simulink library "bluetooth_lib"  (Simulink 6.0)
settings: Solver=ode45  SolverMode=SingleTasking  StartTime=0.0  StopTime=10.0  RelTol=1e-3
undefined symbols (not defined in the file or in its folder): awgn_802_seed, fixed_hop_freq, hop_seed, rate_802_seed
libraries: dspindex x12, commutil2 x12, dspsrcs4 x9, bluetooth_lib x7, dspsigattribs x3, dsparch4 x2, dspsigops x2, commdigbbndfm2 x1, dspstat3 x1, dspbuff3 x1, simulink3 x1
settings Model: Creator=stuartm  LastModifiedBy=mmclerno  ProdHWDeviceType=Specified
settings DataIOCC: SignalLoggingName=logsOut
settings OptimizationCC: BooleanDataType=off
settings DebuggingCC: CheckExecutionContextPreStartOutputMsg=on  CheckExecutionContextRuntimeOutputMsg=on  SolverPrmCheckMsg=none
settings HardwareCC: ProdHWDeviceType=Specified

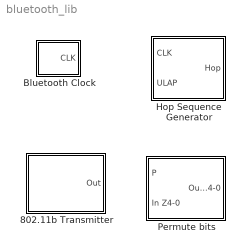
== system bluetooth_lib ==
  802.11b Transmitter : Subsystem  PropExecContextAcrossSSBoundary=on  mask{On=on, rate=200, m=1e-3, v=0, power=0.1, Freq_Number=39, rate_seed=rate_802_seed, awgn_seed=awgn_802_seed}
      mask prompts: On "Turn On 802.11"; rate "Average Rate (1/sec) (999 for constant)"; m "Mean Length (secs)"; v "Length Variance (sec^2)"; Freq_Number "Frequency Number (0-78)"; rate_seed "Rate Seed"; awgn_seed "Noise seed"
      mask init:
      | if On==1
      |    str='On';
      | else
      |   str='Off';
      | end;
      | 
      | adjusted_rate=rate/(1-rate*m); % account for finite packet length reducing rate
      mask Display: disp(['802.11b\nInterferer\n' str])
  Bluetooth Clock : Subsystem  PropExecContextAcrossSSBoundary=on  mask(Bluetooth Clock){Ts=(1/1600)/2}
      mask prompts: Ts "Sample Time"
  Hop Sequence Generator : Subsystem  PropExecContextAcrossSSBoundary=on  mask(Hop Sequence Generator){Hop_Mode=Connection State Hop Sequence, hop_seed=hop_seed, fixed_hop_freq=fixed_hop_freq}
      mask prompts: Hop_Mode "Hop mode"; hop_seed "Hop seed (for white random sequence option)"; fixed_hop_freq "Fixed hop frequency (for fixed option)"
      mask help: Generate a sequence of hop frequencies in the range 0 to 78. Can generate either the connection state hop sequence, a random white sequence, or be fixed.
      mask StyleString: popup(Connection State Hop Sequence|Random White Hop Sequence|Fixed Frequency),edit,edit
  Permute bits : Subsystem  PropExecContextAcrossSSBoundary=on  mask{P=[13 12], First=[1 2], Second=[0 3]}
      mask prompts: P "P bit pair"; First "Pair of bits that first P bit switches"; Second "Pair of bits that second P bit switches"
      mask Display: disp(['P' num2str(P(1)) ': {Z' num2str(First(1)) ',Z' num2str(First(2)) '}\n'  'P' num2str(P(2)) ': {Z' num2str(Second(1)) ',Z' num2str(Second(2)) '}'])

== system bluetooth_lib/802.11b Transmitter ==
  1/100packet resolution : ZeroOrderHold  SampleTime=(1/1600)/100
  22MHz noise in 100MHz signal : Subsystem  TreatAsAtomicUnit=on  PropExecContextAcrossSSBoundary=on
  Buffer to same frame-size as channel : dspbuff3/Buffer  N=62500  V=0  ic=0
  Enable control : Subsystem  PropExecContextAcrossSSBoundary=on
      mask Display:
      | disp('Enable\n
      | Logic')
  Square pulse with Poisson process : Subsystem  PropExecContextAcrossSSBoundary=on  mask(Poisson process){rate=adjusted_rate, m=m, v=v, seed=rate_seed}
      mask prompts: rate "Average Rate (1/sec)"; m "Mean Length"; v "Length Variance"
      mask Display: plot(exp(-(0:.4:3)))
  Out : Outport
  tag scope: Packet_Envelope_802=global
  wires:
  Enable control/1(Out) -> 22MHz noise in 100MHz signal/Enable
  Square pulse with Poisson process/1(hit) -> [Packet_Envelope_802], 1/100packet resolution/1
  1/100packet resolution/1 -> Enable control/1(In)
  Buffer to same frame-size as channel/1 -> Out/1
  22MHz noise in 100MHz signal/1(Out) -> Buffer to same frame-size as channel/1

== system bluetooth_lib/Bluetooth Clock ==
  DSP Constant : dspsrcs4/DSP Constant  Value=1  SampleMode=Discrete  discreteOutput=Sample-based  continuousOutput=Sample-based  sampTime=Ts  framePeriod=Ts  dataType=Inherit from 'Constant value'  wordLen=16  udDataType=sfix(16)  fracBitsMode=Best precision  numFracBits=15  InterpretAs1D=off  Ts=Ts  FramebasedOutput=off
  Delay : dspsigops/Delay  dly_unit=Samples  delay=1  ic_detail=off  dif_ic_for_ch=off  dif_ic_for_dly=off  ic=0  reset_popup=None
  Sum : Sum  Inputs=|++  SaturateOnIntegerOverflow=on  InputSameDT=on
  CLK : Outport
  wires:
  Sum/1 -> Delay/1
  DSP Constant/1 -> Sum/1
  Delay/1 -> Sum/2, CLK/1

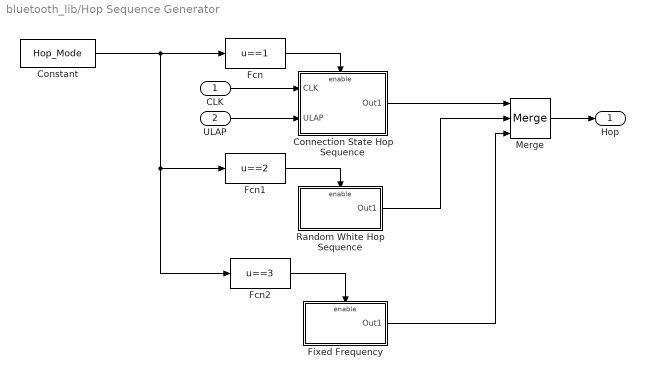
== system bluetooth_lib/Hop Sequence Generator ==
  CLK : Inport  LatchInput=off
  ULAP : Inport  Port=2  LatchInput=off
  Connection State Hop Sequence : Subsystem  TreatAsAtomicUnit=on  PropExecContextAcrossSSBoundary=on
  Constant : Constant  Value=Hop_Mode
  Fcn : Fcn  Expr=u==1
  Fcn1 : Fcn  Expr=u==2
  Fcn2 : Fcn  Expr=u==3
  Fixed Frequency : Subsystem  TreatAsAtomicUnit=on  PropExecContextAcrossSSBoundary=on
  Merge : Merge  Inputs=3
  Random White Hop Sequence : Subsystem  TreatAsAtomicUnit=on  PropExecContextAcrossSSBoundary=on
  Hop : Outport
  wires:
  ULAP/1 -> Connection State Hop Sequence/2(ULAP)
  CLK/1 -> Connection State Hop Sequence/1(CLK)
  Constant/1 -> Fcn/1, Fcn1/1, Fcn2/1
  Merge/1 -> Hop/1
  Connection State Hop Sequence/1(Out1) -> Merge/1
  Random White Hop Sequence/1(Out1) -> Merge/2
  Fixed Frequency/1(Out1) -> Merge/3
  Fcn/1 -> Connection State Hop Sequence/Enable
  Fcn1/1 -> Random White Hop Sequence/Enable
  Fcn2/1 -> Fixed Frequency/Enable

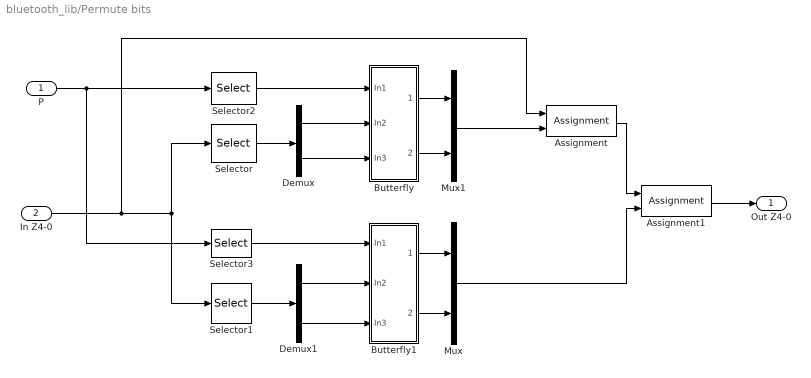
== system bluetooth_lib/Permute bits ==
  P : Inport  LatchInput=off
  In Z4-0 : Inport  Port=2  LatchInput=off
  Assignment : Assignment  Elements=[First(1) First(2)] +1
  Assignment1 : Assignment  Elements=[Second(1) Second(2)] +1
  Butterfly : Subsystem  PropExecContextAcrossSSBoundary=on
  Butterfly1 : Subsystem  PropExecContextAcrossSSBoundary=on
  Demux : Demux  Outputs=2
  Demux1 : Demux  Outputs=2
  Mux : Mux  Inputs=2
  Mux1 : Mux  Inputs=2
  Selector : Selector  Elements=[First(1) First(2)] +1  InputPortWidth=5
  Selector1 : Selector  Elements=[Second(1) Second(2)] +1  InputPortWidth=5
  Selector2 : Selector  Elements=[P(1)] +1  InputPortWidth=14
  Selector3 : Selector  Elements=[P(2)] +1  InputPortWidth=14
  Out Z4-0 : Outport
  wires:
  Demux1/2 -> Butterfly1/3(In3)
  Selector3/1 -> Butterfly1/1(In1)
  Demux/1 -> Butterfly/2(In2)
  Butterfly/1(Out1) -> Mux1/1
  Butterfly1/1(Out1) -> Mux/1
  Butterfly1/2(Out2) -> Mux/2
  Mux/1 -> Assignment1/2
  In Z4-0/1 -> Selector/1, Selector1/1, Assignment/1
  Selector/1 -> Demux/1
  Selector1/1 -> Demux1/1
  Butterfly/2(Out2) -> Mux1/2
  Mux1/1 -> Assignment/2
  Assignment/1 -> Assignment1/1
  Assignment1/1 -> Out Z4-0/1
  Demux/2 -> Butterfly/3(In3)
  Demux1/1 -> Butterfly1/2(In2)
  P/1 -> Selector2/1, Selector3/1
  Selector2/1 -> Butterfly/1(In1)

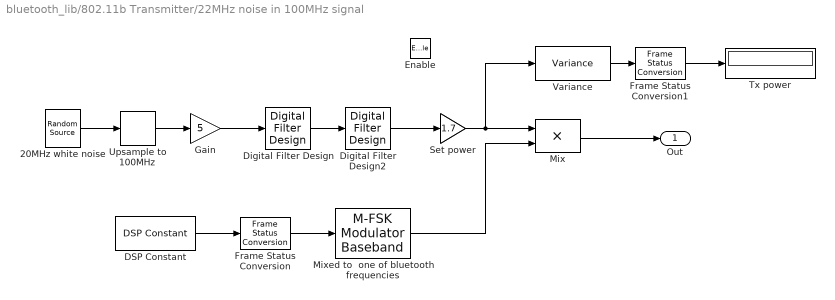
== system bluetooth_lib/802.11b Transmitter/22MHz noise in 100MHz signal ==
  Enable : EnablePort
  20MHz white noise : dspsrcs4/Random Source  SrcType=Gaussian  NormMethod=Ziggurat  CltLength=12  Min=0  Max=1  Mean=0  Var=power  RepMode=Specify seed  rawSeed=awgn_seed  Inherit=off  SampMode=Discrete  SampTime=1/20e6  SampFrame=62500/500  DataType=Double  OutComplex=Complex
  DSP Constant : dspsrcs4/DSP Constant  Value=Freq_Number  SampleMode=Discrete  discreteOutput=Sample-based  continuousOutput=Sample-based  sampTime=.01/1600  framePeriod=.01/1600  dataType=Inherit from 'Constant value'  isSigned=on  wordLen=16  udDataType=sfix(16)  fracBitsMode=Best precision  numFracBits=15  InterpretAs1D=off  Ts=.01/1600  FramebasedOutput=off
  Digital Filter Design : dsparch4/Digital Filter Design
  Digital Filter Design2 : dsparch4/Digital Filter Design
  Frame Status Conversion : dspsigattribs/Frame Status Conversion  growRefPort=off  outframe=Frame-based
  Frame Status Conversion1 : dspsigattribs/Frame Status Conversion  growRefPort=off  outframe=Sample-based
  Gain : Gain  Gain=5  SaturateOnIntegerOverflow=on
  Mix : Product  SaturateOnIntegerOverflow=on  InputSameDT=on
  "Mixed to  one of bluetooth frequencies " : commdigbbndfm2/M-FSK Modulator Baseband  M=79  InType=Integer  Enc=Binary  freqSep=1e6  phaseType=Continuous  numSamp=6.25e4/100
  Set power : Gain  Gain=1.7  SaturateOnIntegerOverflow=on
  Tx power : Display
  Upsample to 100MHz : dspsigops/Upsample  N=5  phase=0  ic=0  mode=Maintain input frame rate
  Variance : dspstat3/Variance  DialogController=dspDDGCreate  DialogControllerArgs=DataTag3  run=off  reset_popup=None  roundingMode=Floor  overflowMode=off
  Out : Outport  OutputWhenDisabled=reset  InitialOutput=0
  wires:
  Digital Filter Design/1 -> Digital Filter Design2/1
  Digital Filter Design2/1 -> Set power/1
  Set power/1 -> Variance/1, Mix/1
  Frame Status Conversion1/1 -> Tx power/1
  Variance/1 -> Frame Status Conversion1/1
  Gain/1 -> Digital Filter Design/1
  DSP Constant/1 -> Frame Status Conversion/1
  "Mixed to  one of bluetooth frequencies "/1 -> Mix/2
  Frame Status Conversion/1 -> "Mixed to  one of bluetooth frequencies "/1
  20MHz white noise/1 -> Upsample to 100MHz/1
  Mix/1 -> Out/1
  Upsample to 100MHz/1 -> Gain/1

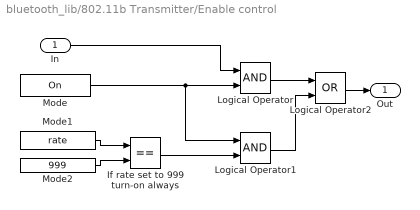
== system bluetooth_lib/802.11b Transmitter/Enable control ==
  In : Inport  LatchInput=off
  If rate set to 999 turn-on always : RelationalOperator  Operator===  InputSameDT=on
  Logical Operator : Logic
  Logical Operator1 : Logic
  Logical Operator2 : Logic  Operator=OR
  Mode : Constant  Value=On
  Mode1 : Constant  Value=rate
  Mode2 : Constant  Value=999
  Out : Outport
  wires:
  Logical Operator2/1 -> Out/1
  In/1 -> Logical Operator/1
  Logical Operator1/1 -> Logical Operator2/2
  Mode/1 -> Logical Operator1/1, Logical Operator/2
  Logical Operator/1 -> Logical Operator2/1
  If rate set to 999 turn-on always/1 -> Logical Operator1/2
  Mode1/1 -> If rate set to 999 turn-on always/1
  Mode2/1 -> If rate set to 999 turn-on always/2

== system bluetooth_lib/802.11b Transmitter/Square pulse with Poisson process ==
  S-Function1 : S-Function  FunctionName=bluetooth_poissonevent  Parameters=adjusted_rate,m,v,seed
  hit : Outport  InitialOutput=0
  wires:
  S-Function1/1 -> hit/1

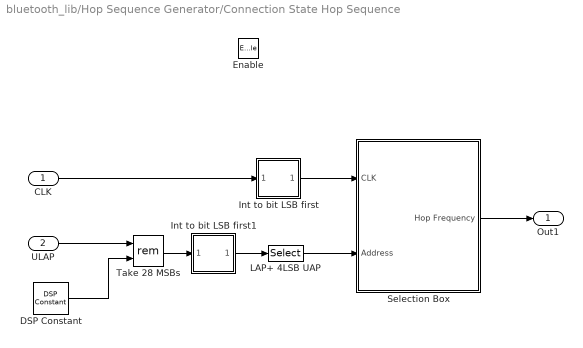
== system bluetooth_lib/Hop Sequence Generator/Connection State Hop Sequence ==
  CLK : Inport  LatchInput=off
  ULAP : Inport  Port=2  LatchInput=off
  Enable : EnablePort
  DSP Constant : dspsrcs4/DSP Constant  Value=2^28  InterpretAs1D=off  SampleMode=Discrete  Ts=(1/1600)/2  FramebasedOutput=off
  Int to bit LSB first : Subsystem  PropExecContextAcrossSSBoundary=on  mask{Numbits=28}
      mask prompts: Numbits "Number of bits"
      mask Display:
      | disp('Int to bit\n
      | LSB first');
  Int to bit LSB first1 : Subsystem  PropExecContextAcrossSSBoundary=on  mask{Numbits=28}
      mask prompts: Numbits "Number of bits"
      mask Display:
      | disp('Int to bit\n
      | LSB first');
  LAP+ 4LSB UAP : Selector  Elements=[0:27] +1  InputPortWidth=28
  Selection Box : Subsystem  PropExecContextAcrossSSBoundary=on
  Take 28 MSBs : Math  Operator=rem  SaturateOnIntegerOverflow=on
  Out1 : Outport
  wires:
  ULAP/1 -> Take 28 MSBs/1
  Take 28 MSBs/1 -> Int to bit LSB first1/1(In1)
  DSP Constant/1 -> Take 28 MSBs/2
  CLK/1 -> Int to bit LSB first/1(In1)
  Int to bit LSB first/1(Out1) -> Selection Box/1(CLK)
  Int to bit LSB first1/1(Out1) -> LAP+ 4LSB UAP/1
  LAP+ 4LSB UAP/1 -> Selection Box/2(Address)
  Selection Box/1(Hop Frequency) -> Out1/1

== system bluetooth_lib/Hop Sequence Generator/Fixed Frequency ==
  Enable : EnablePort
  A fixed hop frequency : dspsrcs4/DSP Constant  Value=fixed_hop_freq  SampleMode=Discrete  discreteOutput=Sample-based (interpret vectors as 1-D)  continuousOutput=Sample-based  sampTime=(1/1600)/2  framePeriod=(1/1600)/2  dataType=Inherit from 'Constant value'  isSigned=on  wordLen=16  udDataType=sfix(16)  fracBitsMode=Best precision  numFracBits=15  InterpretAs1D=on  Ts=(1/1600)/2  FramebasedOutput=off
  Out1 : Outport  InitialOutput=fixed_hop_freq
  wires:
  A fixed hop frequency/1 -> Out1/1

== system bluetooth_lib/Hop Sequence Generator/Random White Hop Sequence ==
  Enable : EnablePort
  Frequency hopping code 1/1600 sec (page 127) : Subsystem  PropExecContextAcrossSSBoundary=on  mask(Random-Integer Generator){mul=79, seed=hop_seed, Ts=(1/1600)/2, frameBased=off, sampPerFrame=1, orient=off}
      mask prompts: mul "M-ary number:"; seed "Initial seed:"; Ts "Sample time:"; frameBased "Frame-based outputs"; sampPerFrame "Samples per frame:"; orient "Interpret vector parameters as 1-D"
      mask help: Generate integers randomly distributed in range [0, M-1], where M is the M-ary number.
      mask init:
      | if (frameBased & sampPerFrame > 1), dsp_sampFrame = sampPerFrame;
      | else dsp_sampFrame = 1; end
      | eStr=commblkrandintsrc2(gcb,'init');
      | if(eStr.ecode==1)
      |     error(eStr.emsg);
      | end
      mask Help: helpview(commbhelp)
      mask CallbackString: |||commblkrandintsrc2(gcb,'cbFrameBased');||commblkrandintsrc2(gcb,'cbOrient');
      mask Display: disp('Random int')
  Out1 : Outport
  wires:
  Frequency hopping code 1/1600 sec (page 127)/1(out_1) -> Out1/1

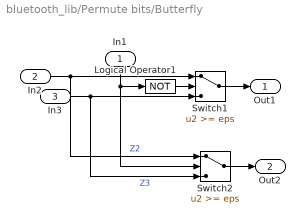
== system bluetooth_lib/Permute bits/Butterfly ==
  In1 : Inport  Orientation=down  LatchInput=off
  In2 : Inport  Port=2  LatchInput=off
  In3 : Inport  Port=3  LatchInput=off
  Logical Operator1 : Logic  Operator=NOT
  Switch1 : Switch  Threshold=eps  SaturateOnIntegerOverflow=on  InputSameDT=on
  Switch2 : Switch  Threshold=eps  SaturateOnIntegerOverflow=on  InputSameDT=on
  Out1 : Outport
  Out2 : Outport  Port=2
  wires:
  Switch2/1 -> Out2/1
  Switch1/1 -> Out1/1
  Logical Operator1/1 -> Switch1/2
  In1/1 -> Switch2/2, Logical Operator1/1
  In3/1 -> Switch1/3, Switch2/3  "Z3"
  In2/1 -> Switch1/1, Switch2/1  "Z2"

== system bluetooth_lib/Permute bits/Butterfly1 ==
  In1 : Inport  Orientation=down  LatchInput=off
  In2 : Inport  Port=2  LatchInput=off
  In3 : Inport  Port=3  LatchInput=off
  Logical Operator1 : Logic  Operator=NOT
  Switch1 : Switch  Threshold=eps  SaturateOnIntegerOverflow=on  InputSameDT=on
  Switch2 : Switch  Threshold=eps  SaturateOnIntegerOverflow=on  InputSameDT=on
  Out1 : Outport
  Out2 : Outport  Port=2
  wires:
  In2/1 -> Switch2/1, Switch1/1  "Z2"
  In3/1 -> Switch2/3, Switch1/3  "Z3"
  In1/1 -> Logical Operator1/1, Switch2/2
  Logical Operator1/1 -> Switch1/2
  Switch1/1 -> Out1/1
  Switch2/1 -> Out2/1

== system bluetooth_lib/Hop Sequence Generator/Connection State Hop Sequence/Int to bit LSB first ==
  In1 : Inport  LatchInput=off
  Flip : dspindex/Flip  dim=Columns
  Integer to Bit Converter3 : commutil2/Integer to Bit Converter  nbits=Numbits
  Out1 : Outport
  wires:
  Integer to Bit Converter3/1 -> Flip/1
  Flip/1 -> Out1/1
  In1/1 -> Integer to Bit Converter3/1

== system bluetooth_lib/Hop Sequence Generator/Connection State Hop Sequence/Int to bit LSB first1 ==
  In1 : Inport  LatchInput=off
  Flip : dspindex/Flip  dim=Columns
  Integer to Bit Converter3 : commutil2/Integer to Bit Converter  nbits=Numbits
  Out1 : Outport
  wires:
  In1/1 -> Integer to Bit Converter3/1
  Flip/1 -> Out1/1
  Integer to Bit Converter3/1 -> Flip/1

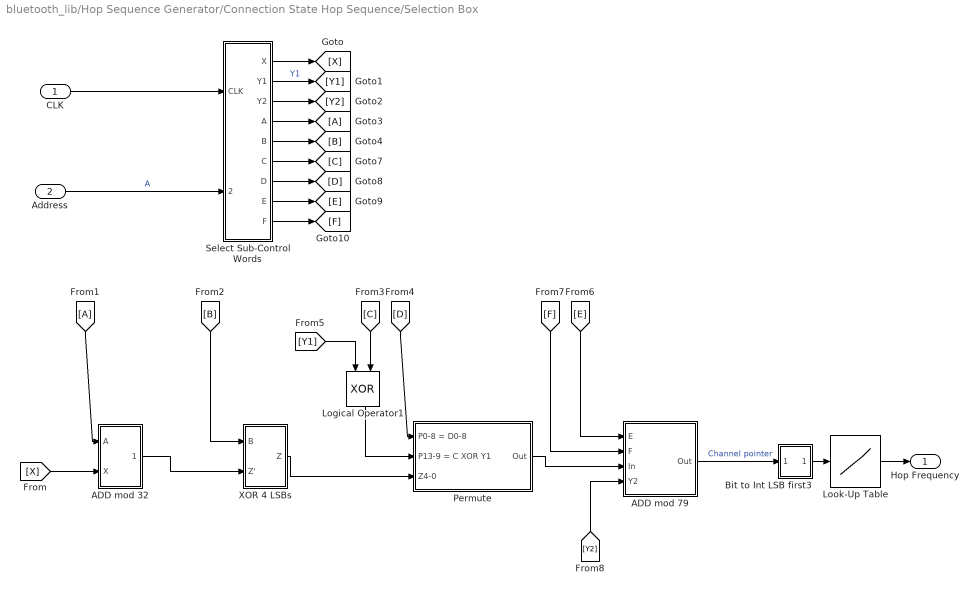
== system bluetooth_lib/Hop Sequence Generator/Connection State Hop Sequence/Selection Box ==
  CLK : Inport  LatchInput=off
  Address : Inport  Port=2  LatchInput=off
  ADD mod 32 : Subsystem  PropExecContextAcrossSSBoundary=on
  ADD mod 79 : Subsystem  PropExecContextAcrossSSBoundary=on
  Bit to Int LSB first3 : Subsystem  PropExecContextAcrossSSBoundary=on  mask{Numbits=7}
      mask prompts: Numbits "Number of bits"
      mask Display:
      | disp('Bit to Int\n
      | LSB first');
  Logical Operator1 : Logic  Orientation=down  Operator=XOR
  Look-Up Table : Lookup  DialogController=Simulink.DDGSource  InputValues=0:78  OutputValues=[0:2:78 1:2:77]  SaturateOnIntegerOverflow=on
  Permute : Subsystem  PropExecContextAcrossSSBoundary=on
  Select Sub-Control Words : Subsystem  PropExecContextAcrossSSBoundary=on
  XOR 4 LSBs : Subsystem  PropExecContextAcrossSSBoundary=on
  Hop Frequency : Outport
  wires:
  [A] -> ADD mod 32/1(A)
  [B] -> XOR 4 LSBs/1(B)
  Logical Operator1/1 -> Permute/2(P13-9 = C XOR Y1)
  [D] -> Permute/1(P0-8 = D0-8)
  Permute/1(Out) -> ADD mod 79/3(In)
  [C] -> Logical Operator1/2
  [Y1] -> Logical Operator1/1
  [E] -> ADD mod 79/1(E)
  [F] -> ADD mod 79/2(F)
  [Y2] -> ADD mod 79/4(Y2)
  ADD mod 79/1(Out) -> Bit to Int LSB first3/1(In1)  "Channel pointer"
  XOR 4 LSBs/1(Z) -> Permute/3(Z4-0)
  Look-Up Table/1 -> Hop Frequency/1
  CLK/1 -> Select Sub-Control Words/1(CLK)
  Select Sub-Control Words/1(X) -> [X]
  Select Sub-Control Words/3(Y2) -> [Y2]
  Address/1 -> Select Sub-Control Words/2(Address)  "A"
  Select Sub-Control Words/4(A) -> [A]
  Select Sub-Control Words/5(B) -> [B]
  Select Sub-Control Words/6(C) -> [C]
  Select Sub-Control Words/7(D) -> [D]
  Select Sub-Control Words/8(E) -> [E]
  Select Sub-Control Words/9(F) -> [F]
  Select Sub-Control Words/2(Y1) -> [Y1]  "Y1"
  [X] -> ADD mod 32/2(X)
  ADD mod 32/1(Out1) -> XOR 4 LSBs/2(Z')
  Bit to Int LSB first3/1(Out1) -> Look-Up Table/1

== system bluetooth_lib/Hop Sequence Generator/Random White Hop Sequence/Frequency hopping code 1/1600 sec (page 127) ==
  Frame Status Conversion : dspsigattribs/Frame Status Conversion  growRefPort=off  outframe=Sample-based
  Random Source : dspsrcs4/Random Source  SrcType=Uniform  Min=-1+eps  Max=mul-1  Mean=0  Var=1  RepMode=Specify seed  Seed=seed  Inherit=off  SampMode=Discrete  SampTime=Ts  SampFrame=dsp_sampFrame  OutComplex=Real
  Reshape : simulink3/Signals & Systems/Reshape  OutputDimensionality=1-D array  OutputDimensions=[sampPerFrame,max([length(mul), length(seed)])]
  Rounding Function : Rounding  Operator=ceil
  out_1 : Outport  InitialOutput=0
  wires:
  Frame Status Conversion/1 -> Reshape/1
  Random Source/1 -> Rounding Function/1
  Reshape/1 -> out_1/1
  Rounding Function/1 -> Frame Status Conversion/1

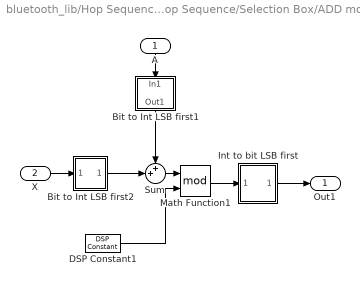
== system bluetooth_lib/Hop Sequence Generator/Connection State Hop Sequence/Selection Box/ADD mod 32 ==
  A : Inport  Orientation=down  LatchInput=off
  X : Inport  Port=2  LatchInput=off
  Bit to Int LSB first1 : Subsystem  Orientation=down  PropExecContextAcrossSSBoundary=on  mask{Numbits=5}
      mask prompts: Numbits "Number of bits"
      mask Display:
      | disp('Bit to Int\n
      | LSB first');
  Bit to Int LSB first2 : Subsystem  PropExecContextAcrossSSBoundary=on  mask{Numbits=5}
      mask prompts: Numbits "Number of bits"
      mask Display:
      | disp('Bit to Int\n
      | LSB first');
  DSP Constant1 : dspsrcs4/DSP Constant  Value=32  InterpretAs1D=off  SampleMode=Discrete  Ts=(1/1600)/2  FramebasedOutput=off
  Int to bit LSB first : Subsystem  PropExecContextAcrossSSBoundary=on  mask{Numbits=5}
      mask prompts: Numbits "Number of bits"
      mask Display:
      | disp('Int to bit\n
      | LSB first');
  Math Function1 : Math  Operator=mod  SaturateOnIntegerOverflow=on
  Sum : Sum  Inputs=++|  SaturateOnIntegerOverflow=on  InputSameDT=on
  Out1 : Outport
  wires:
  Bit to Int LSB first2/1(Out1) -> Sum/2
  Bit to Int LSB first1/1(Out1) -> Sum/1
  Math Function1/1 -> Int to bit LSB first/1(In1)
  Sum/1 -> Math Function1/1
  DSP Constant1/1 -> Math Function1/2
  A/1 -> Bit to Int LSB first1/1(In1)
  X/1 -> Bit to Int LSB first2/1(In1)
  Int to bit LSB first/1(Out1) -> Out1/1

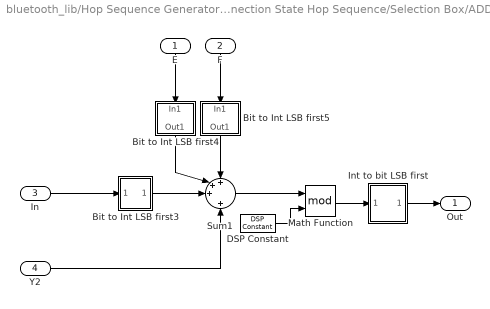
== system bluetooth_lib/Hop Sequence Generator/Connection State Hop Sequence/Selection Box/ADD mod 79 ==
  E : Inport  Orientation=down  LatchInput=off
  F : Inport  Orientation=down  Port=2  LatchInput=off
  In : Inport  Port=3  LatchInput=off
  Y2 : Inport  Port=4  LatchInput=off
  Bit to Int LSB first3 : Subsystem  PropExecContextAcrossSSBoundary=on  mask{Numbits=5}
      mask prompts: Numbits "Number of bits"
      mask Display:
      | disp('Bit to Int\n
      | LSB first');
  Bit to Int LSB first4 : Subsystem  Orientation=down  PropExecContextAcrossSSBoundary=on  mask{Numbits=7}
      mask prompts: Numbits "Number of bits"
      mask Display:
      | disp('Bit to Int\n
      | LSB first');
  Bit to Int LSB first5 : Subsystem  Orientation=down  PropExecContextAcrossSSBoundary=on  mask{Numbits=7}
      mask prompts: Numbits "Number of bits"
      mask Display:
      | disp('Bit to Int\n
      | LSB first');
  DSP Constant : dspsrcs4/DSP Constant  Value=79  InterpretAs1D=off  SampleMode=Discrete  Ts=(1/1600)/2  FramebasedOutput=off
  Int to bit LSB first : Subsystem  PropExecContextAcrossSSBoundary=on  mask{Numbits=7}
      mask prompts: Numbits "Number of bits"
      mask Display:
      | disp('Int to bit\n
      | LSB first');
  Math Function : Math  Operator=mod  SaturateOnIntegerOverflow=on
  Sum1 : Sum  Inputs=+++|+  SaturateOnIntegerOverflow=on  InputSameDT=on
  Out : Outport
  wires:
  Bit to Int LSB first5/1(Out1) -> Sum1/1
  Bit to Int LSB first4/1(Out1) -> Sum1/2
  Sum1/1 -> Math Function/1
  DSP Constant/1 -> Math Function/2
  Bit to Int LSB first3/1(Out1) -> Sum1/3
  E/1 -> Bit to Int LSB first4/1(In1)
  F/1 -> Bit to Int LSB first5/1(In1)
  In/1 -> Bit to Int LSB first3/1(In1)
  Math Function/1 -> Int to bit LSB first/1(In1)
  Y2/1 -> Sum1/4
  Int to bit LSB first/1(Out1) -> Out/1

== system bluetooth_lib/Hop Sequence Generator/Connection State Hop Sequence/Selection Box/Bit to Int LSB first3 ==
  In1 : Inport  LatchInput=off
  Bit to Integer Converter5 : commutil2/Bit to Integer Converter  nbits=Numbits
  Flip1 : dspindex/Flip  dim=Columns
  Out1 : Outport
  wires:
  Flip1/1 -> Bit to Integer Converter5/1
  Bit to Integer Converter5/1 -> Out1/1
  In1/1 -> Flip1/1

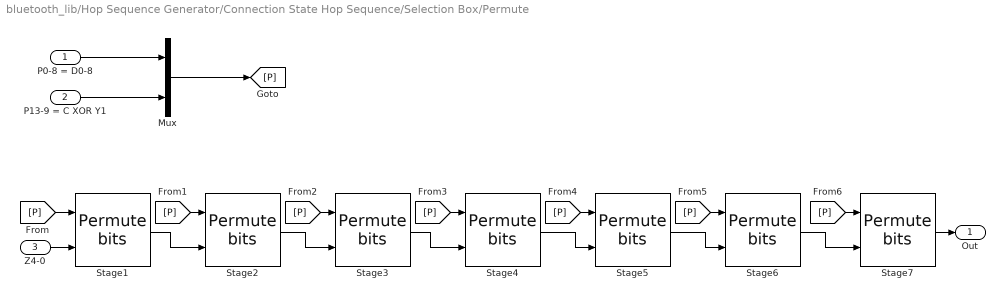
== system bluetooth_lib/Hop Sequence Generator/Connection State Hop Sequence/Selection Box/Permute ==
  P0-8 = D0-8 : Inport  LatchInput=off
  P13-9 = C XOR Y1 : Inport  Port=2  LatchInput=off
  Z4-0 : Inport  Port=3  LatchInput=off
  Mux : Mux  Inputs=2
  Stage1 : bluetooth_lib/Permute bits  P=[13 12]  First=[1 2]  Second=[0 3]
  Stage2 : bluetooth_lib/Permute bits  P=[11 10]  First=[1 3]  Second=[2 4]
  Stage3 : bluetooth_lib/Permute bits  P=[9 8]  First=[0 3]  Second=[1 4]
  Stage4 : bluetooth_lib/Permute bits  P=[7 6]  First=[3 4]  Second=[0 2]
  Stage5 : bluetooth_lib/Permute bits  P=[5 4]  First=[1 3]  Second=[0 4]
  Stage6 : bluetooth_lib/Permute bits  P=[3 2]  First=[3 4]  Second=[1 2]
  Stage7 : bluetooth_lib/Permute bits  P=[1 0]  First=[2 3]  Second=[0 1]
  Out : Outport
  wires:
  Z4-0/1 -> Stage1/2
  Stage1/1 -> Stage2/2
  Mux/1 -> [P]
  [P] -> Stage1/1
  Stage2/1 -> Stage3/2
  [P] -> Stage3/1
  Stage3/1 -> Stage4/2
  [P] -> Stage4/1
  [P] -> Stage5/1
  Stage4/1 -> Stage5/2
  [P] -> Stage6/1
  Stage5/1 -> Stage6/2
  [P] -> Stage7/1
  Stage6/1 -> Stage7/2
  Stage7/1 -> Out/1
  P13-9 = C XOR Y1/1 -> Mux/2
  P0-8 = D0-8/1 -> Mux/1
  [P] -> Stage2/1

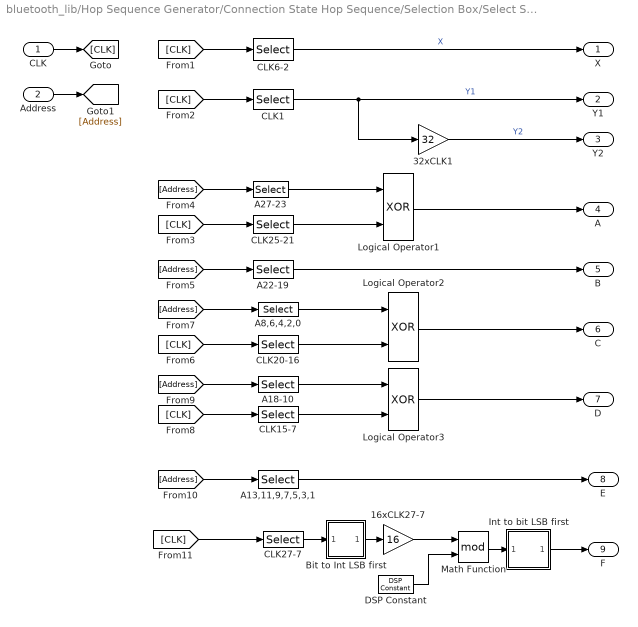
== system bluetooth_lib/Hop Sequence Generator/Connection State Hop Sequence/Selection Box/Select Sub-Control Words ==
  CLK : Inport  LatchInput=off
  Address : Inport  Port=2  LatchInput=off
  16xCLK27-7 : Gain  Gain=16  SaturateOnIntegerOverflow=on
  32xCLK1 : Gain  Gain=32  SaturateOnIntegerOverflow=on
  A13,11,9,7,5,3,1 : Selector  Elements=[1 3 5 7 9 11 13] +1  InputPortWidth=28
  A18-10 : Selector  Elements=[10:18] +1  InputPortWidth=28
  A22-19 : Selector  Elements=[19:22] +1  InputPortWidth=28
  A27-23 : Selector  Elements=[23:27] +1  InputPortWidth=28
  A8,6,4,2,0 : Selector  Elements=[0 2 4 6 8] +1  InputPortWidth=28
  Bit to Int LSB first : Subsystem  PropExecContextAcrossSSBoundary=on  mask{Numbits=21}
      mask prompts: Numbits "Number of bits"
      mask Display:
      | disp('Bit to Int\n
      | LSB first');
  CLK1 : Selector  Elements=[1] +1  InputPortWidth=28
  CLK15-7 : Selector  Elements=[7:15] +1  InputPortWidth=28
  CLK20-16 : Selector  Elements=[16:20] +1  InputPortWidth=28
  CLK25-21 : Selector  Elements=[21:25] +1  InputPortWidth=28
  CLK27-7 : Selector  Elements=[7:27] +1  InputPortWidth=28
  CLK6-2 : Selector  Elements=[2:6] +1  InputPortWidth=28
  DSP Constant : dspsrcs4/DSP Constant  Value=79  InterpretAs1D=off  SampleMode=Discrete  Ts=(1/1600)/2  FramebasedOutput=off
  Int to bit LSB first : Subsystem  PropExecContextAcrossSSBoundary=on  mask{Numbits=7}
      mask prompts: Numbits "Number of bits"
      mask Display:
      | disp('Int to bit\n
      | LSB first');
  Logical Operator1 : Logic  Operator=XOR
  Logical Operator2 : Logic  Operator=XOR
  Logical Operator3 : Logic  Operator=XOR
  Math Function : Math  Operator=mod  SaturateOnIntegerOverflow=on
  X : Outport
  Y1 : Outport  Port=2
  Y2 : Outport  Port=3
  A : Outport  Port=4
  B : Outport  Port=5
  C : Outport  Port=6
  D : Outport  Port=7
  E : Outport  Port=8
  F : Outport  Port=9
  wires:
  CLK1/1 -> 32xCLK1/1, Y1/1  "Y1"
  [CLK] -> CLK6-2/1
  [CLK] -> CLK1/1
  [CLK] -> CLK25-21/1
  [Address] -> A27-23/1
  [Address] -> A22-19/1
  [CLK] -> CLK20-16/1
  CLK20-16/1 -> Logical Operator2/2
  A27-23/1 -> Logical Operator1/1
  CLK25-21/1 -> Logical Operator1/2
  [Address] -> A8,6,4,2,0/1
  A8,6,4,2,0/1 -> Logical Operator2/1
  [CLK] -> CLK15-7/1
  CLK15-7/1 -> Logical Operator3/2
  [Address] -> A18-10/1
  A18-10/1 -> Logical Operator3/1
  [Address] -> A13,11,9,7,5,3,1/1
  [CLK] -> CLK27-7/1
  CLK27-7/1 -> Bit to Int LSB first/1(In1)
  Bit to Int LSB first/1(Out1) -> 16xCLK27-7/1
  16xCLK27-7/1 -> Math Function/1
  DSP Constant/1 -> Math Function/2
  Math Function/1 -> Int to bit LSB first/1(In1)
  CLK6-2/1 -> X/1  "X"
  32xCLK1/1 -> Y2/1  "Y2"
  Logical Operator1/1 -> A/1
  A22-19/1 -> B/1
  Logical Operator2/1 -> C/1
  Logical Operator3/1 -> D/1
  A13,11,9,7,5,3,1/1 -> E/1
  Int to bit LSB first/1(Out1) -> F/1
  CLK/1 -> [CLK]
  Address/1 -> [Address]

== system bluetooth_lib/Hop Sequence Generator/Connection State Hop Sequence/Selection Box/XOR 4 LSBs ==
  B : Inport  LatchInput=off
  Z' : Inport  Port=2  LatchInput=off
  Logical Operator2 : Logic  Operator=XOR
  Mux : Mux  Inputs=2
  Z'3-0 : Selector  Elements=[0:3] +1  InputPortWidth=5
  Z'4 : Selector  Elements=4 +1  InputPortWidth=5
  Z : Outport
  wires:
  Z'3-0/1 -> Logical Operator2/2
  Z'/1 -> Z'4/1, Z'3-0/1
  B/1 -> Logical Operator2/1
  Mux/1 -> Z/1
  Logical Operator2/1 -> Mux/1
  Z'4/1 -> Mux/2

== system bluetooth_lib/Hop Sequence Generator/Connection State Hop Sequence/Selection Box/ADD mod 32/Bit to Int LSB first1 ==
  In1 : Inport  LatchInput=off
  Bit to Integer Converter5 : commutil2/Bit to Integer Converter  nbits=Numbits
  Flip1 : dspindex/Flip  dim=Columns
  Out1 : Outport
  wires:
  Flip1/1 -> Bit to Integer Converter5/1
  Bit to Integer Converter5/1 -> Out1/1
  In1/1 -> Flip1/1

== system bluetooth_lib/Hop Sequence Generator/Connection State Hop Sequence/Selection Box/ADD mod 32/Bit to Int LSB first2 ==
  In1 : Inport  LatchInput=off
  Bit to Integer Converter5 : commutil2/Bit to Integer Converter  nbits=Numbits
  Flip1 : dspindex/Flip  dim=Columns
  Out1 : Outport
  wires:
  In1/1 -> Flip1/1
  Bit to Integer Converter5/1 -> Out1/1
  Flip1/1 -> Bit to Integer Converter5/1

== system bluetooth_lib/Hop Sequence Generator/Connection State Hop Sequence/Selection Box/ADD mod 32/Int to bit LSB first ==
  In1 : Inport  LatchInput=off
  Flip : dspindex/Flip  dim=Columns
  Integer to Bit Converter3 : commutil2/Integer to Bit Converter  nbits=Numbits
  Out1 : Outport
  wires:
  Integer to Bit Converter3/1 -> Flip/1
  Flip/1 -> Out1/1
  In1/1 -> Integer to Bit Converter3/1

== system bluetooth_lib/Hop Sequence Generator/Connection State Hop Sequence/Selection Box/ADD mod 79/Bit to Int LSB first3 ==
  In1 : Inport  LatchInput=off
  Bit to Integer Converter5 : commutil2/Bit to Integer Converter  nbits=Numbits
  Flip1 : dspindex/Flip  dim=Columns
  Out1 : Outport
  wires:
  Flip1/1 -> Bit to Integer Converter5/1
  Bit to Integer Converter5/1 -> Out1/1
  In1/1 -> Flip1/1

== system bluetooth_lib/Hop Sequence Generator/Connection State Hop Sequence/Selection Box/ADD mod 79/Bit to Int LSB first4 ==
  In1 : Inport  LatchInput=off
  Bit to Integer Converter5 : commutil2/Bit to Integer Converter  nbits=Numbits
  Flip1 : dspindex/Flip  dim=Columns
  Out1 : Outport
  wires:
  In1/1 -> Flip1/1
  Bit to Integer Converter5/1 -> Out1/1
  Flip1/1 -> Bit to Integer Converter5/1

== system bluetooth_lib/Hop Sequence Generator/Connection State Hop Sequence/Selection Box/ADD mod 79/Bit to Int LSB first5 ==
  In1 : Inport  LatchInput=off
  Bit to Integer Converter5 : commutil2/Bit to Integer Converter  nbits=Numbits
  Flip1 : dspindex/Flip  dim=Columns
  Out1 : Outport
  wires:
  Flip1/1 -> Bit to Integer Converter5/1
  Bit to Integer Converter5/1 -> Out1/1
  In1/1 -> Flip1/1

== system bluetooth_lib/Hop Sequence Generator/Connection State Hop Sequence/Selection Box/ADD mod 79/Int to bit LSB first ==
  In1 : Inport  LatchInput=off
  Flip : dspindex/Flip  dim=Columns
  Integer to Bit Converter3 : commutil2/Integer to Bit Converter  nbits=Numbits
  Out1 : Outport
  wires:
  Integer to Bit Converter3/1 -> Flip/1
  Flip/1 -> Out1/1
  In1/1 -> Integer to Bit Converter3/1

== system bluetooth_lib/Hop Sequence Generator/Connection State Hop Sequence/Selection Box/Select Sub-Control Words/Bit to Int LSB first ==
  In1 : Inport  LatchInput=off
  Bit to Integer Converter5 : commutil2/Bit to Integer Converter  nbits=Numbits
  Flip1 : dspindex/Flip  dim=Columns
  Out1 : Outport
  wires:
  Flip1/1 -> Bit to Integer Converter5/1
  Bit to Integer Converter5/1 -> Out1/1
  In1/1 -> Flip1/1

== system bluetooth_lib/Hop Sequence Generator/Connection State Hop Sequence/Selection Box/Select Sub-Control Words/Int to bit LSB first ==
  In1 : Inport  LatchInput=off
  Flip : dspindex/Flip  dim=Columns
  Integer to Bit Converter3 : commutil2/Integer to Bit Converter  nbits=Numbits
  Out1 : Outport
  wires:
  Integer to Bit Converter3/1 -> Flip/1
  Flip/1 -> Out1/1
  In1/1 -> Integer to Bit Converter3/1
